simulink model "Tetris"  (R2023a)
settings: Solver=VariableStepAuto  StartTime=0.0  StopTime=inf  RelTol=1e-3  EnableMultiTasking=on
libraries: Miscellaneous x183, Byte_Multiplexers_Lib x77, Tetris_Lib x34, simulink_extras x11, Counters_Lib x7, Arithmetic_Operations_Lib x5, Word_Multiplexers_Lib x5, Decoders_Lib x4, Memory_Blocks_Lib x3, Bit_Multiplexers_Lib x2, dspobslib x1
(part 2 of 3)

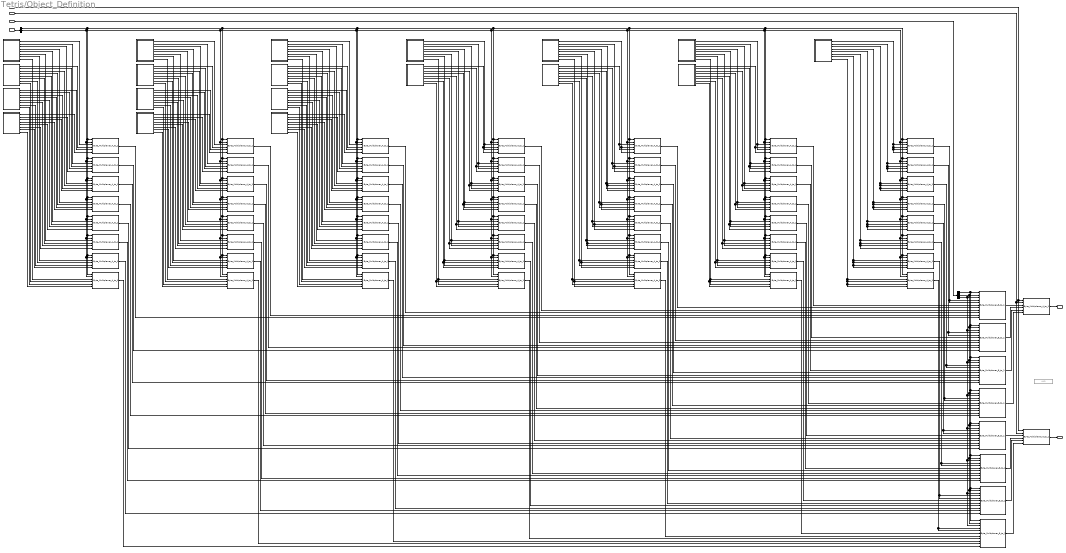
== system Tetris/Object_Definition ==
  Addr_1(1b) : Inport
  Addr_0(1b) : Inport  Port=2
  Shape(1B) : Inport  Port=3
  Angle(1B) : Inport  Port=4
  Bus Selector1 : BusSelector  OutputSignals=signal6,signal7,signal8
  Bus Selector2 : BusSelector  OutputSignals=signal7,signal8
  Byte_Multiplexer_4_to_1(X) : Byte_Multiplexers_Lib/Byte_Multiplexers_Lib/Byte_Multiplexer_4_to_1  SystemSampleTime=-1  VariantActivationTime=update diagram  Latency=0  AutoFrameSizeCalculation=off
  Byte_Multiplexer_4_to_1(Y) : Byte_Multiplexers_Lib/Byte_Multiplexers_Lib/Byte_Multiplexer_4_to_1  SystemSampleTime=-1  VariantActivationTime=update diagram  Latency=0  AutoFrameSizeCalculation=off
  I-shape (0deg) : Subsystem
  I-shape (90deg) : Subsystem
  L1-shape (0deg) : Subsystem
  L1-shape (180deg) : Subsystem
  L1-shape (270deg) : Subsystem
  L1-shape (90deg) : Subsystem
  L2-shape (0deg) : Subsystem
  L2-shape (180deg) : Subsystem
  L2-shape (270deg) : Subsystem
  L2-shape (90deg) : Subsystem
  Logical Operator1 : Logic  Commented=on  Inputs=12  IconShape=distinctive  AllPortsSameDT=off  OutDataTypeStr=boolean
  O-shape : Subsystem
  Select_Angle_I(X0) : Byte_Multiplexers_Lib/Byte_Multiplexers_Lib/Byte_Multiplexer_4_to_1  SystemSampleTime=-1  VariantActivationTime=update diagram  Latency=0  AutoFrameSizeCalculation=off
  Select_Angle_I(X1) : Byte_Multiplexers_Lib/Byte_Multiplexers_Lib/Byte_Multiplexer_4_to_1  SystemSampleTime=-1  VariantActivationTime=update diagram  Latency=0  AutoFrameSizeCalculation=off
  Select_Angle_I(X2) : Byte_Multiplexers_Lib/Byte_Multiplexers_Lib/Byte_Multiplexer_4_to_1  SystemSampleTime=-1  VariantActivationTime=update diagram  Latency=0  AutoFrameSizeCalculation=off
  Select_Angle_I(X3) : Byte_Multiplexers_Lib/Byte_Multiplexers_Lib/Byte_Multiplexer_4_to_1  SystemSampleTime=-1  VariantActivationTime=update diagram  Latency=0  AutoFrameSizeCalculation=off
  Select_Angle_I(Y0) : Byte_Multiplexers_Lib/Byte_Multiplexers_Lib/Byte_Multiplexer_4_to_1  SystemSampleTime=-1  VariantActivationTime=update diagram  Latency=0  AutoFrameSizeCalculation=off
  Select_Angle_I(Y1) : Byte_Multiplexers_Lib/Byte_Multiplexers_Lib/Byte_Multiplexer_4_to_1  SystemSampleTime=-1  VariantActivationTime=update diagram  Latency=0  AutoFrameSizeCalculation=off
  Select_Angle_I(Y2) : Byte_Multiplexers_Lib/Byte_Multiplexers_Lib/Byte_Multiplexer_4_to_1  SystemSampleTime=-1  VariantActivationTime=update diagram  Latency=0  AutoFrameSizeCalculation=off
  Select_Angle_I(Y3) : Byte_Multiplexers_Lib/Byte_Multiplexers_Lib/Byte_Multiplexer_4_to_1  SystemSampleTime=-1  VariantActivationTime=update diagram  Latency=0  AutoFrameSizeCalculation=off
  Select_Angle_L1(X0) : Byte_Multiplexers_Lib/Byte_Multiplexers_Lib/Byte_Multiplexer_4_to_1  SystemSampleTime=-1  VariantActivationTime=update diagram  Latency=0  AutoFrameSizeCalculation=off
  Select_Angle_L1(X1) : Byte_Multiplexers_Lib/Byte_Multiplexers_Lib/Byte_Multiplexer_4_to_1  SystemSampleTime=-1  VariantActivationTime=update diagram  Latency=0  AutoFrameSizeCalculation=off
  Select_Angle_L1(X2) : Byte_Multiplexers_Lib/Byte_Multiplexers_Lib/Byte_Multiplexer_4_to_1  SystemSampleTime=-1  VariantActivationTime=update diagram  Latency=0  AutoFrameSizeCalculation=off
  Select_Angle_L1(X3) : Byte_Multiplexers_Lib/Byte_Multiplexers_Lib/Byte_Multiplexer_4_to_1  SystemSampleTime=-1  VariantActivationTime=update diagram  Latency=0  AutoFrameSizeCalculation=off
  Select_Angle_L1(Y0) : Byte_Multiplexers_Lib/Byte_Multiplexers_Lib/Byte_Multiplexer_4_to_1  SystemSampleTime=-1  VariantActivationTime=update diagram  Latency=0  AutoFrameSizeCalculation=off
  Select_Angle_L1(Y1) : Byte_Multiplexers_Lib/Byte_Multiplexers_Lib/Byte_Multiplexer_4_to_1  SystemSampleTime=-1  VariantActivationTime=update diagram  Latency=0  AutoFrameSizeCalculation=off
  Select_Angle_L1(Y2) : Byte_Multiplexers_Lib/Byte_Multiplexers_Lib/Byte_Multiplexer_4_to_1  SystemSampleTime=-1  VariantActivationTime=update diagram  Latency=0  AutoFrameSizeCalculation=off
  Select_Angle_L1(Y3) : Byte_Multiplexers_Lib/Byte_Multiplexers_Lib/Byte_Multiplexer_4_to_1  SystemSampleTime=-1  VariantActivationTime=update diagram  Latency=0  AutoFrameSizeCalculation=off
  Select_Angle_L2(X0) : Byte_Multiplexers_Lib/Byte_Multiplexers_Lib/Byte_Multiplexer_4_to_1  SystemSampleTime=-1  VariantActivationTime=update diagram  Latency=0  AutoFrameSizeCalculation=off
  Select_Angle_L2(X1) : Byte_Multiplexers_Lib/Byte_Multiplexers_Lib/Byte_Multiplexer_4_to_1  SystemSampleTime=-1  VariantActivationTime=update diagram  Latency=0  AutoFrameSizeCalculation=off
  Select_Angle_L2(X2) : Byte_Multiplexers_Lib/Byte_Multiplexers_Lib/Byte_Multiplexer_4_to_1  SystemSampleTime=-1  VariantActivationTime=update diagram  Latency=0  AutoFrameSizeCalculation=off
  Select_Angle_L2(X3) : Byte_Multiplexers_Lib/Byte_Multiplexers_Lib/Byte_Multiplexer_4_to_1  SystemSampleTime=-1  VariantActivationTime=update diagram  Latency=0  AutoFrameSizeCalculation=off
  Select_Angle_L2(Y0) : Byte_Multiplexers_Lib/Byte_Multiplexers_Lib/Byte_Multiplexer_4_to_1  SystemSampleTime=-1  VariantActivationTime=update diagram  Latency=0  AutoFrameSizeCalculation=off
  Select_Angle_L2(Y1) : Byte_Multiplexers_Lib/Byte_Multiplexers_Lib/Byte_Multiplexer_4_to_1  SystemSampleTime=-1  VariantActivationTime=update diagram  Latency=0  AutoFrameSizeCalculation=off
  Select_Angle_L2(Y2) : Byte_Multiplexers_Lib/Byte_Multiplexers_Lib/Byte_Multiplexer_4_to_1  SystemSampleTime=-1  VariantActivationTime=update diagram  Latency=0  AutoFrameSizeCalculation=off
  Select_Angle_L2(Y3) : Byte_Multiplexers_Lib/Byte_Multiplexers_Lib/Byte_Multiplexer_4_to_1  SystemSampleTime=-1  VariantActivationTime=update diagram  Latency=0  AutoFrameSizeCalculation=off
  Select_Angle_O(X0) : Byte_Multiplexers_Lib/Byte_Multiplexers_Lib/Byte_Multiplexer_4_to_1  SystemSampleTime=-1  VariantActivationTime=update diagram  Latency=0  AutoFrameSizeCalculation=off
  Select_Angle_O(X1) : Byte_Multiplexers_Lib/Byte_Multiplexers_Lib/Byte_Multiplexer_4_to_1  SystemSampleTime=-1  VariantActivationTime=update diagram  Latency=0  AutoFrameSizeCalculation=off
  Select_Angle_O(X2) : Byte_Multiplexers_Lib/Byte_Multiplexers_Lib/Byte_Multiplexer_4_to_1  SystemSampleTime=-1  VariantActivationTime=update diagram  Latency=0  AutoFrameSizeCalculation=off
  Select_Angle_O(X3) : Byte_Multiplexers_Lib/Byte_Multiplexers_Lib/Byte_Multiplexer_4_to_1  SystemSampleTime=-1  VariantActivationTime=update diagram  Latency=0  AutoFrameSizeCalculation=off
  Select_Angle_O(Y0) : Byte_Multiplexers_Lib/Byte_Multiplexers_Lib/Byte_Multiplexer_4_to_1  SystemSampleTime=-1  VariantActivationTime=update diagram  Latency=0  AutoFrameSizeCalculation=off
  Select_Angle_O(Y1) : Byte_Multiplexers_Lib/Byte_Multiplexers_Lib/Byte_Multiplexer_4_to_1  SystemSampleTime=-1  VariantActivationTime=update diagram  Latency=0  AutoFrameSizeCalculation=off
  Select_Angle_O(Y2) : Byte_Multiplexers_Lib/Byte_Multiplexers_Lib/Byte_Multiplexer_4_to_1  SystemSampleTime=-1  VariantActivationTime=update diagram  Latency=0  AutoFrameSizeCalculation=off
  Select_Angle_O(Y3) : Byte_Multiplexers_Lib/Byte_Multiplexers_Lib/Byte_Multiplexer_4_to_1  SystemSampleTime=-1  VariantActivationTime=update diagram  Latency=0  AutoFrameSizeCalculation=off
  Select_Angle_T(X0) : Byte_Multiplexers_Lib/Byte_Multiplexers_Lib/Byte_Multiplexer_4_to_1  SystemSampleTime=-1  VariantActivationTime=update diagram  Latency=0  AutoFrameSizeCalculation=off
  Select_Angle_T(X1) : Byte_Multiplexers_Lib/Byte_Multiplexers_Lib/Byte_Multiplexer_4_to_1  SystemSampleTime=-1  VariantActivationTime=update diagram  Latency=0  AutoFrameSizeCalculation=off
  Select_Angle_T(X2) : Byte_Multiplexers_Lib/Byte_Multiplexers_Lib/Byte_Multiplexer_4_to_1  SystemSampleTime=-1  VariantActivationTime=update diagram  Latency=0  AutoFrameSizeCalculation=off
  Select_Angle_T(X3) : Byte_Multiplexers_Lib/Byte_Multiplexers_Lib/Byte_Multiplexer_4_to_1  SystemSampleTime=-1  VariantActivationTime=update diagram  Latency=0  AutoFrameSizeCalculation=off
  Select_Angle_T(Y0) : Byte_Multiplexers_Lib/Byte_Multiplexers_Lib/Byte_Multiplexer_4_to_1  SystemSampleTime=-1  VariantActivationTime=update diagram  Latency=0  AutoFrameSizeCalculation=off
  Select_Angle_T(Y1) : Byte_Multiplexers_Lib/Byte_Multiplexers_Lib/Byte_Multiplexer_4_to_1  SystemSampleTime=-1  VariantActivationTime=update diagram  Latency=0  AutoFrameSizeCalculation=off
  Select_Angle_T(Y2) : Byte_Multiplexers_Lib/Byte_Multiplexers_Lib/Byte_Multiplexer_4_to_1  SystemSampleTime=-1  VariantActivationTime=update diagram  Latency=0  AutoFrameSizeCalculation=off
  Select_Angle_T(Y3) : Byte_Multiplexers_Lib/Byte_Multiplexers_Lib/Byte_Multiplexer_4_to_1  SystemSampleTime=-1  VariantActivationTime=update diagram  Latency=0  AutoFrameSizeCalculation=off
  Select_Angle_Z1(X0) : Byte_Multiplexers_Lib/Byte_Multiplexers_Lib/Byte_Multiplexer_4_to_1  SystemSampleTime=-1  VariantActivationTime=update diagram  Latency=0  AutoFrameSizeCalculation=off
  Select_Angle_Z1(X1) : Byte_Multiplexers_Lib/Byte_Multiplexers_Lib/Byte_Multiplexer_4_to_1  SystemSampleTime=-1  VariantActivationTime=update diagram  Latency=0  AutoFrameSizeCalculation=off
  Select_Angle_Z1(X2) : Byte_Multiplexers_Lib/Byte_Multiplexers_Lib/Byte_Multiplexer_4_to_1  SystemSampleTime=-1  VariantActivationTime=update diagram  Latency=0  AutoFrameSizeCalculation=off
  Select_Angle_Z1(X3) : Byte_Multiplexers_Lib/Byte_Multiplexers_Lib/Byte_Multiplexer_4_to_1  SystemSampleTime=-1  VariantActivationTime=update diagram  Latency=0  AutoFrameSizeCalculation=off
  Select_Angle_Z1(Y0) : Byte_Multiplexers_Lib/Byte_Multiplexers_Lib/Byte_Multiplexer_4_to_1  SystemSampleTime=-1  VariantActivationTime=update diagram  Latency=0  AutoFrameSizeCalculation=off
  Select_Angle_Z1(Y1) : Byte_Multiplexers_Lib/Byte_Multiplexers_Lib/Byte_Multiplexer_4_to_1  SystemSampleTime=-1  VariantActivationTime=update diagram  Latency=0  AutoFrameSizeCalculation=off
  Select_Angle_Z1(Y2) : Byte_Multiplexers_Lib/Byte_Multiplexers_Lib/Byte_Multiplexer_4_to_1  SystemSampleTime=-1  VariantActivationTime=update diagram  Latency=0  AutoFrameSizeCalculation=off
  Select_Angle_Z1(Y3) : Byte_Multiplexers_Lib/Byte_Multiplexers_Lib/Byte_Multiplexer_4_to_1  SystemSampleTime=-1  VariantActivationTime=update diagram  Latency=0  AutoFrameSizeCalculation=off
  Select_Angle_Z2(X0) : Byte_Multiplexers_Lib/Byte_Multiplexers_Lib/Byte_Multiplexer_4_to_1  SystemSampleTime=-1  VariantActivationTime=update diagram  Latency=0  AutoFrameSizeCalculation=off
  Select_Angle_Z2(X1) : Byte_Multiplexers_Lib/Byte_Multiplexers_Lib/Byte_Multiplexer_4_to_1  SystemSampleTime=-1  VariantActivationTime=update diagram  Latency=0  AutoFrameSizeCalculation=off
  Select_Angle_Z2(X2) : Byte_Multiplexers_Lib/Byte_Multiplexers_Lib/Byte_Multiplexer_4_to_1  SystemSampleTime=-1  VariantActivationTime=update diagram  Latency=0  AutoFrameSizeCalculation=off
  Select_Angle_Z2(X3) : Byte_Multiplexers_Lib/Byte_Multiplexers_Lib/Byte_Multiplexer_4_to_1  SystemSampleTime=-1  VariantActivationTime=update diagram  Latency=0  AutoFrameSizeCalculation=off
  Select_Angle_Z2(Y0) : Byte_Multiplexers_Lib/Byte_Multiplexers_Lib/Byte_Multiplexer_4_to_1  SystemSampleTime=-1  VariantActivationTime=update diagram  Latency=0  AutoFrameSizeCalculation=off
  Select_Angle_Z2(Y1) : Byte_Multiplexers_Lib/Byte_Multiplexers_Lib/Byte_Multiplexer_4_to_1  SystemSampleTime=-1  VariantActivationTime=update diagram  Latency=0  AutoFrameSizeCalculation=off
  Select_Angle_Z2(Y2) : Byte_Multiplexers_Lib/Byte_Multiplexers_Lib/Byte_Multiplexer_4_to_1  SystemSampleTime=-1  VariantActivationTime=update diagram  Latency=0  AutoFrameSizeCalculation=off
  Select_Angle_Z2(Y3) : Byte_Multiplexers_Lib/Byte_Multiplexers_Lib/Byte_Multiplexer_4_to_1  SystemSampleTime=-1  VariantActivationTime=update diagram  Latency=0  AutoFrameSizeCalculation=off
  Select_Shape(X0) : Byte_Multiplexers_Lib/Byte_Multiplexers_Lib/Byte_Multiplexer_8_to_1  SystemSampleTime=-1  VariantActivationTime=update diagram  Latency=0  AutoFrameSizeCalculation=off
  Select_Shape(X1) : Byte_Multiplexers_Lib/Byte_Multiplexers_Lib/Byte_Multiplexer_8_to_1  SystemSampleTime=-1  VariantActivationTime=update diagram  Latency=0  AutoFrameSizeCalculation=off
  Select_Shape(X2) : Byte_Multiplexers_Lib/Byte_Multiplexers_Lib/Byte_Multiplexer_8_to_1  SystemSampleTime=-1  VariantActivationTime=update diagram  Latency=0  AutoFrameSizeCalculation=off
  Select_Shape(X3) : Byte_Multiplexers_Lib/Byte_Multiplexers_Lib/Byte_Multiplexer_8_to_1  SystemSampleTime=-1  VariantActivationTime=update diagram  Latency=0  AutoFrameSizeCalculation=off
  Select_Shape(Y0) : Byte_Multiplexers_Lib/Byte_Multiplexers_Lib/Byte_Multiplexer_8_to_1  SystemSampleTime=-1  VariantActivationTime=update diagram  Latency=0  AutoFrameSizeCalculation=off
  Select_Shape(Y1) : Byte_Multiplexers_Lib/Byte_Multiplexers_Lib/Byte_Multiplexer_8_to_1  SystemSampleTime=-1  VariantActivationTime=update diagram  Latency=0  AutoFrameSizeCalculation=off
  Select_Shape(Y2) : Byte_Multiplexers_Lib/Byte_Multiplexers_Lib/Byte_Multiplexer_8_to_1  SystemSampleTime=-1  VariantActivationTime=update diagram  Latency=0  AutoFrameSizeCalculation=off
  Select_Shape(Y3) : Byte_Multiplexers_Lib/Byte_Multiplexers_Lib/Byte_Multiplexer_8_to_1  SystemSampleTime=-1  VariantActivationTime=update diagram  Latency=0  AutoFrameSizeCalculation=off
  T-shape (0deg) : Subsystem
  T-shape (180deg) : Subsystem
  T-shape (270deg) : Subsystem
  T-shape (90deg) : Subsystem
  Z1-shape (0deg) : Subsystem
  Z1-shape (90deg) : Subsystem
  Z2-shape (0deg) : Subsystem
  Z2-shape (90deg) : Subsystem
  X(1B) : Outport
  Y(1B) : Outport  Port=2
  wires:
  L2-shape (0deg)/1(X0(1B)) -> Select_Angle_L2(X3)/3
  L2-shape (90deg)/1(X0(1B)) -> Select_Angle_L2(X3)/4
  L2-shape (180deg)/1(X0(1B)) -> Select_Angle_L2(X3)/5
  L2-shape (270deg)/1(X0(1B)) -> Select_Angle_L2(X3)/6
  L2-shape (0deg)/2(X1(1B)) -> Select_Angle_L2(X2)/3
  L2-shape (90deg)/2(X1(1B)) -> Select_Angle_L2(X2)/4
  L2-shape (180deg)/2(X1(1B)) -> Select_Angle_L2(X2)/5
  L2-shape (270deg)/2(X1(1B)) -> Select_Angle_L2(X2)/6
  L2-shape (0deg)/3(X2(1B)) -> Select_Angle_L2(X1)/3
  L2-shape (90deg)/3(X2(1B)) -> Select_Angle_L2(X1)/4
  L2-shape (180deg)/3(X2(1B)) -> Select_Angle_L2(X1)/5
  L2-shape (270deg)/3(X2(1B)) -> Select_Angle_L2(X1)/6
  L2-shape (0deg)/4(X3(1B)) -> Select_Angle_L2(X0)/3
  L2-shape (90deg)/4(X3(1B)) -> Select_Angle_L2(X0)/4
  L2-shape (180deg)/4(X3(1B)) -> Select_Angle_L2(X0)/5
  L2-shape (270deg)/4(X3(1B)) -> Select_Angle_L2(X0)/6
  L2-shape (0deg)/5(Y0(1B)) -> Select_Angle_L2(Y3)/3
  L2-shape (90deg)/5(Y0(1B)) -> Select_Angle_L2(Y3)/4
  L2-shape (180deg)/5(Y0(1B)) -> Select_Angle_L2(Y3)/5
  L2-shape (270deg)/5(Y0(1B)) -> Select_Angle_L2(Y3)/6
  L2-shape (0deg)/6(Y1(1B)) -> Select_Angle_L2(Y2)/3
  L2-shape (90deg)/6(Y1(1B)) -> Select_Angle_L2(Y2)/4
  L2-shape (180deg)/6(Y1(1B)) -> Select_Angle_L2(Y2)/5
  L2-shape (270deg)/6(Y1(1B)) -> Select_Angle_L2(Y2)/6
  L2-shape (0deg)/7(Y2(1B)) -> Select_Angle_L2(Y1)/3
  L2-shape (90deg)/7(Y2(1B)) -> Select_Angle_L2(Y1)/4
  L2-shape (180deg)/7(Y2(1B)) -> Select_Angle_L2(Y1)/5
  L2-shape (270deg)/7(Y2(1B)) -> Select_Angle_L2(Y1)/6
  L2-shape (0deg)/8(Y3(1B)) -> Select_Angle_L2(Y0)/3
  L2-shape (90deg)/8(Y3(1B)) -> Select_Angle_L2(Y0)/4
  L2-shape (180deg)/8(Y3(1B)) -> Select_Angle_L2(Y0)/5
  L2-shape (270deg)/8(Y3(1B)) -> Select_Angle_L2(Y0)/6
  Angle(1B)/1 -> Bus Selector2/1
  L1-shape (270deg)/4(X3(1B)) -> Select_Angle_L1(X0)/6
  L1-shape (180deg)/4(X3(1B)) -> Select_Angle_L1(X0)/5
  L1-shape (270deg)/6(Y1(1B)) -> Select_Angle_L1(Y2)/6
  L1-shape (180deg)/5(Y0(1B)) -> Select_Angle_L1(Y3)/5
  L1-shape (90deg)/8(Y3(1B)) -> Select_Angle_L1(Y0)/4
  L1-shape (180deg)/1(X0(1B)) -> Select_Angle_L1(X3)/5
  L1-shape (270deg)/5(Y0(1B)) -> Select_Angle_L1(Y3)/6
  L1-shape (90deg)/6(Y1(1B)) -> Select_Angle_L1(Y2)/4
  L1-shape (0deg)/2(X1(1B)) -> Select_Angle_L1(X2)/3
  L1-shape (90deg)/2(X1(1B)) -> Select_Angle_L1(X2)/4
  L1-shape (270deg)/8(Y3(1B)) -> Select_Angle_L1(Y0)/6
  L1-shape (180deg)/6(Y1(1B)) -> Select_Angle_L1(Y2)/5
  L1-shape (0deg)/6(Y1(1B)) -> Select_Angle_L1(Y2)/3
  L1-shape (90deg)/7(Y2(1B)) -> Select_Angle_L1(Y1)/4
  L1-shape (90deg)/3(X2(1B)) -> Select_Angle_L1(X1)/4
  L1-shape (180deg)/3(X2(1B)) -> Select_Angle_L1(X1)/5
  L1-shape (0deg)/1(X0(1B)) -> Select_Angle_L1(X3)/3
  L1-shape (0deg)/7(Y2(1B)) -> Select_Angle_L1(Y1)/3
  L1-shape (0deg)/3(X2(1B)) -> Select_Angle_L1(X1)/3
  L1-shape (0deg)/4(X3(1B)) -> Select_Angle_L1(X0)/3
  L1-shape (270deg)/2(X1(1B)) -> Select_Angle_L1(X2)/6
  L1-shape (90deg)/5(Y0(1B)) -> Select_Angle_L1(Y3)/4
  L1-shape (180deg)/7(Y2(1B)) -> Select_Angle_L1(Y1)/5
  L1-shape (90deg)/1(X0(1B)) -> Select_Angle_L1(X3)/4
  L1-shape (180deg)/8(Y3(1B)) -> Select_Angle_L1(Y0)/5
  L1-shape (270deg)/7(Y2(1B)) -> Select_Angle_L1(Y1)/6
  L1-shape (270deg)/1(X0(1B)) -> Select_Angle_L1(X3)/6
  L1-shape (0deg)/5(Y0(1B)) -> Select_Angle_L1(Y3)/3
  L1-shape (270deg)/3(X2(1B)) -> Select_Angle_L1(X1)/6
  L1-shape (180deg)/2(X1(1B)) -> Select_Angle_L1(X2)/5
  L1-shape (0deg)/8(Y3(1B)) -> Select_Angle_L1(Y0)/3
  L1-shape (90deg)/4(X3(1B)) -> Select_Angle_L1(X0)/4
  T-shape (90deg)/1(X0(1B)) -> Select_Angle_T(X3)/4
  T-shape (90deg)/5(Y0(1B)) -> Select_Angle_T(Y3)/4
  T-shape (90deg)/7(Y2(1B)) -> Select_Angle_T(Y1)/4
  T-shape (90deg)/6(Y1(1B)) -> Select_Angle_T(Y2)/4
  T-shape (180deg)/8(Y3(1B)) -> Select_Angle_T(Y0)/5
  T-shape (180deg)/6(Y1(1B)) -> Select_Angle_T(Y2)/5
  T-shape (90deg)/4(X3(1B)) -> Select_Angle_T(X0)/4
  T-shape (180deg)/7(Y2(1B)) -> Select_Angle_T(Y1)/5
  T-shape (180deg)/4(X3(1B)) -> Select_Angle_T(X0)/5
  T-shape (180deg)/1(X0(1B)) -> Select_Angle_T(X3)/5
  T-shape (180deg)/3(X2(1B)) -> Select_Angle_T(X1)/5
  T-shape (90deg)/2(X1(1B)) -> Select_Angle_T(X2)/4
  T-shape (180deg)/5(Y0(1B)) -> Select_Angle_T(Y3)/5
  T-shape (270deg)/1(X0(1B)) -> Select_Angle_T(X3)/6
  T-shape (270deg)/5(Y0(1B)) -> Select_Angle_T(Y3)/6
  T-shape (270deg)/7(Y2(1B)) -> Select_Angle_T(Y1)/6
  T-shape (270deg)/4(X3(1B)) -> Select_Angle_T(X0)/6
  T-shape (270deg)/3(X2(1B)) -> Select_Angle_T(X1)/6
  T-shape (270deg)/2(X1(1B)) -> Select_Angle_T(X2)/6
  T-shape (270deg)/8(Y3(1B)) -> Select_Angle_T(Y0)/6
  T-shape (270deg)/6(Y1(1B)) -> Select_Angle_T(Y2)/6
  T-shape (0deg)/1(X0(1B)) -> Select_Angle_T(X3)/3
  T-shape (180deg)/2(X1(1B)) -> Select_Angle_T(X2)/5
  T-shape (0deg)/8(Y3(1B)) -> Select_Angle_T(Y0)/3
  T-shape (90deg)/8(Y3(1B)) -> Select_Angle_T(Y0)/4
  T-shape (0deg)/6(Y1(1B)) -> Select_Angle_T(Y2)/3
  T-shape (0deg)/3(X2(1B)) -> Select_Angle_T(X1)/3
  T-shape (0deg)/4(X3(1B)) -> Select_Angle_T(X0)/3
  T-shape (90deg)/3(X2(1B)) -> Select_Angle_T(X1)/4
  T-shape (0deg)/2(X1(1B)) -> Select_Angle_T(X2)/3
  T-shape (0deg)/5(Y0(1B)) -> Select_Angle_T(Y3)/3
  T-shape (0deg)/7(Y2(1B)) -> Select_Angle_T(Y1)/3
  Z2-shape (0deg)/8(Y3(1B)) -> Select_Angle_Z2(Y0)/5, Select_Angle_Z2(Y0)/3
  Z2-shape (0deg)/6(Y1(1B)) -> Select_Angle_Z2(Y2)/5, Select_Angle_Z2(Y2)/3
  Z2-shape (0deg)/7(Y2(1B)) -> Select_Angle_Z2(Y1)/5, Select_Angle_Z2(Y1)/3
  Z2-shape (0deg)/4(X3(1B)) -> Select_Angle_Z2(X0)/5, Select_Angle_Z2(X0)/3
  Z2-shape (0deg)/1(X0(1B)) -> Select_Angle_Z2(X3)/5, Select_Angle_Z2(X3)/3
  Z2-shape (0deg)/3(X2(1B)) -> Select_Angle_Z2(X1)/5, Select_Angle_Z2(X1)/3
  Z2-shape (0deg)/5(Y0(1B)) -> Select_Angle_Z2(Y3)/5, Select_Angle_Z2(Y3)/3
  Z2-shape (90deg)/1(X0(1B)) -> Select_Angle_Z2(X3)/6, Select_Angle_Z2(X3)/4
  Z2-shape (90deg)/5(Y0(1B)) -> Select_Angle_Z2(Y3)/6, Select_Angle_Z2(Y3)/4
  Z2-shape (90deg)/7(Y2(1B)) -> Select_Angle_Z2(Y1)/6, Select_Angle_Z2(Y1)/4
  Z2-shape (90deg)/4(X3(1B)) -> Select_Angle_Z2(X0)/6, Select_Angle_Z2(X0)/4
  Z2-shape (90deg)/3(X2(1B)) -> Select_Angle_Z2(X1)/6, Select_Angle_Z2(X1)/4
  Z2-shape (90deg)/2(X1(1B)) -> Select_Angle_Z2(X2)/6, Select_Angle_Z2(X2)/4
  Z2-shape (90deg)/8(Y3(1B)) -> Select_Angle_Z2(Y0)/6, Select_Angle_Z2(Y0)/4
  Z2-shape (90deg)/6(Y1(1B)) -> Select_Angle_Z2(Y2)/6, Select_Angle_Z2(Y2)/4
  Z2-shape (0deg)/2(X1(1B)) -> Select_Angle_Z2(X2)/5, Select_Angle_Z2(X2)/3
  Z1-shape (90deg)/7(Y1(1B)) -> Select_Angle_Z1(Y1)/5, Select_Angle_Z1(Y1)/3
  Z1-shape (90deg)/2(X2(1B)) -> Select_Angle_Z1(X2)/5, Select_Angle_Z1(X2)/3
  Z1-shape (90deg)/4(X0(1B)) -> Select_Angle_Z1(X0)/5, Select_Angle_Z1(X0)/3
  Z1-shape (90deg)/3(X1(1B)) -> Select_Angle_Z1(X1)/5, Select_Angle_Z1(X1)/3
  Z1-shape (90deg)/6(Y2(1B)) -> Select_Angle_Z1(Y2)/5, Select_Angle_Z1(Y2)/3
  Z1-shape (90deg)/5(Y3(1B)) -> Select_Angle_Z1(Y3)/5, Select_Angle_Z1(Y3)/3
  Z1-shape (90deg)/1(X3(1B)) -> Select_Angle_Z1(X3)/5, Select_Angle_Z1(X3)/3
  Z1-shape (0deg)/6(Y2(1B)) -> Select_Angle_Z1(Y2)/6, Select_Angle_Z1(Y2)/4
  Z1-shape (0deg)/4(X0(1B)) -> Select_Angle_Z1(X0)/6, Select_Angle_Z1(X0)/4
  Z1-shape (0deg)/1(X3(1B)) -> Select_Angle_Z1(X3)/6, Select_Angle_Z1(X3)/4
  Z1-shape (0deg)/5(Y3(1B)) -> Select_Angle_Z1(Y3)/6, Select_Angle_Z1(Y3)/4
  Z1-shape (90deg)/8(Y0(1B)) -> Select_Angle_Z1(Y0)/5, Select_Angle_Z1(Y0)/3
  Z1-shape (0deg)/2(X2(1B)) -> Select_Angle_Z1(X2)/4, Select_Angle_Z1(X2)/6
  Z1-shape (0deg)/3(X1(1B)) -> Select_Angle_Z1(X1)/6, Select_Angle_Z1(X1)/4
  Z1-shape (0deg)/8(Y0(1B)) -> Select_Angle_Z1(Y0)/6, Select_Angle_Z1(Y0)/4
  Z1-shape (0deg)/7(Y1(1B)) -> Select_Angle_Z1(Y1)/6, Select_Angle_Z1(Y1)/4
  I-shape (90deg)/7(Y2(1B)) -> Select_Angle_I(Y1)/6, Select_Angle_I(Y1)/4
  I-shape (90deg)/2(X1(1B)) -> Select_Angle_I(X2)/6, Select_Angle_I(X2)/4
  I-shape (90deg)/4(X3(1B)) -> Select_Angle_I(X0)/6, Select_Angle_I(X0)/4
  I-shape (90deg)/3(X2(1B)) -> Select_Angle_I(X1)/6, Select_Angle_I(X1)/4
  I-shape (90deg)/6(Y1(1B)) -> Select_Angle_I(Y2)/6, Select_Angle_I(Y2)/4
  I-shape (90deg)/5(Y0(1B)) -> Select_Angle_I(Y3)/6, Select_Angle_I(Y3)/4
  I-shape (90deg)/1(X0(1B)) -> Select_Angle_I(X3)/6, Select_Angle_I(X3)/4
  I-shape (0deg)/6(Y1(1B)) -> Select_Angle_I(Y2)/5, Select_Angle_I(Y2)/3
  I-shape (0deg)/4(X3(1B)) -> Select_Angle_I(X0)/5, Select_Angle_I(X0)/3
  I-shape (0deg)/1(X0(1B)) -> Select_Angle_I(X3)/5, Select_Angle_I(X3)/3
  I-shape (0deg)/5(Y0(1B)) -> Select_Angle_I(Y3)/5, Select_Angle_I(Y3)/3
  I-shape (90deg)/8(Y3(1B)) -> Select_Angle_I(Y0)/6, Select_Angle_I(Y0)/4
  I-shape (0deg)/2(X1(1B)) -> Select_Angle_I(X2)/5, Select_Angle_I(X2)/3
  I-shape (0deg)/3(X2(1B)) -> Select_Angle_I(X1)/5, Select_Angle_I(X1)/3
  I-shape (0deg)/8(Y3(1B)) -> Select_Angle_I(Y0)/5, Select_Angle_I(Y0)/3
  I-shape (0deg)/7(Y2(1B)) -> Select_Angle_I(Y1)/5, Select_Angle_I(Y1)/3
  O-shape/7(Y2(1B)) -> Select_Angle_O(Y1)/5, Select_Angle_O(Y1)/6, Select_Angle_O(Y1)/4, Select_Angle_O(Y1)/3
  O-shape/2(X1(1B)) -> Select_Angle_O(X2)/5, Select_Angle_O(X2)/6, Select_Angle_O(X2)/4, Select_Angle_O(X2)/3
  O-shape/4(X3(1B)) -> Select_Angle_O(X0)/5, Select_Angle_O(X0)/6, Select_Angle_O(X0)/4, Select_Angle_O(X0)/3
  O-shape/3(X2(1B)) -> Select_Angle_O(X1)/5, Select_Angle_O(X1)/6, Select_Angle_O(X1)/4, Select_Angle_O(X1)/3
  O-shape/6(Y1(1B)) -> Select_Angle_O(Y2)/6, Select_Angle_O(Y2)/5, Select_Angle_O(Y2)/4, Select_Angle_O(Y2)/3
  O-shape/5(Y0(1B)) -> Select_Angle_O(Y3)/5, Select_Angle_O(Y3)/6, Select_Angle_O(Y3)/4, Select_Angle_O(Y3)/3
  O-shape/1(X0(1B)) -> Select_Angle_O(X3)/5, Select_Angle_O(X3)/6, Select_Angle_O(X3)/4, Select_Angle_O(X3)/3
  Bus Selector2/1 -> Select_Angle_L2(Y0)/1, Select_Angle_L2(Y1)/1, Select_Angle_L2(Y2)/1, Select_Angle_L2(Y3)/1, Select_Angle_L2(X0)/1, Select_Angle_L2(X1)/1, Select_Angle_L2(X2)/1, Select_Angle_L2(X3)/1, Select_Angle_Z1(Y0)/1, Select_Angle_Z1(Y1)/1, Select_Angle_Z1(Y2)/1, Select_Angle_Z1(Y3)/1, Select_Angle_Z1(X0)/1, Select_Angle_Z1(X1)/1, Select_Angle_Z1(X2)/1, Select_Angle_Z1(X3)/1, Select_Angle_O(Y0)/1, Select_Angle_O(Y1)/1, Select_Angle_O(Y2)/1, Select_Angle_O(Y3)/1, Select_Angle_O(X0)/1, Select_Angle_O(X1)/1, Select_Angle_O(X2)/1, Select_Angle_O(X3)/1, Select_Angle_I(Y0)/1, Select_Angle_I(Y1)/1, Select_Angle_I(Y2)/1, Select_Angle_I(Y3)/1, Select_Angle_I(X0)/1, Select_Angle_I(X1)/1, Select_Angle_I(X2)/1, Select_Angle_I(X3)/1, Select_Angle_Z2(Y0)/1, Select_Angle_Z2(Y1)/1, Select_Angle_Z2(Y2)/1, Select_Angle_Z2(Y3)/1, Select_Angle_Z2(X0)/1, Select_Angle_Z2(X1)/1, Select_Angle_Z2(X2)/1, Select_Angle_Z2(X3)/1, Select_Angle_T(Y0)/1, Select_Angle_T(Y1)/1, Select_Angle_T(Y2)/1, Select_Angle_T(Y3)/1, Select_Angle_T(X0)/1, Select_Angle_T(X1)/1, Select_Angle_T(X2)/1, Select_Angle_T(X3)/1, Select_Angle_L1(Y0)/1, Select_Angle_L1(Y1)/1, Select_Angle_L1(Y2)/1, Select_Angle_L1(Y3)/1, Select_Angle_L1(X0)/1, Select_Angle_L1(X1)/1, Select_Angle_L1(X2)/1, Select_Angle_L1(X3)/1  "<signal7>"
  Bus Selector2/2 -> Select_Angle_L2(Y0)/2, Select_Angle_L2(Y1)/2, Select_Angle_L2(Y2)/2, Select_Angle_L2(Y3)/2, Select_Angle_L2(X0)/2, Select_Angle_L2(X1)/2, Select_Angle_L2(X2)/2, Select_Angle_L2(X3)/2, Select_Angle_Z1(Y0)/2, Select_Angle_Z1(Y1)/2, Select_Angle_Z1(Y2)/2, Select_Angle_Z1(Y3)/2, Select_Angle_Z1(X0)/2, Select_Angle_Z1(X1)/2, Select_Angle_Z1(X2)/2, Select_Angle_Z1(X3)/2, Select_Angle_O(Y0)/2, Select_Angle_O(Y1)/2, Select_Angle_O(Y2)/2, Select_Angle_O(Y3)/2, Select_Angle_O(X0)/2, Select_Angle_O(X1)/2, Select_Angle_O(X2)/2, Select_Angle_O(X3)/2, Select_Angle_I(Y0)/2, Select_Angle_I(Y1)/2, Select_Angle_I(Y2)/2, Select_Angle_I(Y3)/2, Select_Angle_I(X0)/2, Select_Angle_I(X1)/2, Select_Angle_I(X2)/2, Select_Angle_I(X3)/2, Select_Angle_Z2(Y0)/2, Select_Angle_Z2(Y1)/2, Select_Angle_Z2(Y2)/2, Select_Angle_Z2(Y3)/2, Select_Angle_Z2(X0)/2, Select_Angle_Z2(X1)/2, Select_Angle_Z2(X2)/2, Select_Angle_Z2(X3)/2, Select_Angle_T(Y0)/2, Select_Angle_T(Y1)/2, Select_Angle_T(Y2)/2, Select_Angle_T(Y3)/2, Select_Angle_T(X0)/2, Select_Angle_T(X1)/2, Select_Angle_T(X2)/2, Select_Angle_T(X3)/2, Select_Angle_L1(Y0)/2, Select_Angle_L1(Y1)/2, Select_Angle_L1(Y2)/2, Select_Angle_L1(Y3)/2, Select_Angle_L1(X0)/2, Select_Angle_L1(X1)/2, Select_Angle_L1(X2)/2, Select_Angle_L1(X3)/2  "<signal8>"
  O-shape/8(Y3(1B)) -> Select_Angle_O(Y0)/5, Select_Angle_O(Y0)/6, Select_Angle_O(Y0)/4, Select_Angle_O(Y0)/3
  Select_Angle_O(X3)/1 -> Select_Shape(X3)/4, Select_Shape(X3)/5
  Select_Angle_I(X3)/1 -> Select_Shape(X3)/6
  Select_Angle_Z1(X3)/1 -> Select_Shape(X3)/7
  Select_Angle_Z2(X3)/1 -> Select_Shape(X3)/8
  Select_Angle_T(X3)/1 -> Select_Shape(X3)/9
  Select_Angle_L1(X3)/1 -> Select_Shape(X3)/10
  Select_Angle_L2(X3)/1 -> Select_Shape(X3)/11
  Select_Angle_L2(X2)/1 -> Select_Shape(X2)/11
  Select_Angle_L2(X1)/1 -> Select_Shape(X1)/11
  Select_Angle_L2(X0)/1 -> Select_Shape(X0)/11
  Select_Angle_L2(Y3)/1 -> Select_Shape(Y3)/11
  Select_Angle_L2(Y2)/1 -> Select_Shape(Y2)/11
  Select_Angle_L2(Y1)/1 -> Select_Shape(Y1)/11
  Select_Angle_L2(Y0)/1 -> Select_Shape(Y0)/11
  Select_Angle_L1(X2)/1 -> Select_Shape(X2)/10
  Select_Angle_L1(X1)/1 -> Select_Shape(X1)/10
  Select_Angle_L1(X0)/1 -> Select_Shape(X0)/10
  Select_Angle_L1(Y3)/1 -> Select_Shape(Y3)/10
  Select_Angle_L1(Y2)/1 -> Select_Shape(Y2)/10
  Select_Angle_L1(Y1)/1 -> Select_Shape(Y1)/10
  Select_Angle_L1(Y0)/1 -> Select_Shape(Y0)/10
  Select_Angle_T(X2)/1 -> Select_Shape(X2)/9
  Select_Angle_T(X1)/1 -> Select_Shape(X1)/9
  Select_Angle_T(X0)/1 -> Select_Shape(X0)/9
  Select_Angle_T(Y3)/1 -> Select_Shape(Y3)/9
  Select_Angle_T(Y2)/1 -> Select_Shape(Y2)/9
  Select_Angle_T(Y1)/1 -> Select_Shape(Y1)/9
  Select_Angle_T(Y0)/1 -> Select_Shape(Y0)/9
  Select_Angle_Z2(X2)/1 -> Select_Shape(X2)/8
  Select_Angle_Z2(X1)/1 -> Select_Shape(X1)/8
  Select_Angle_Z2(X0)/1 -> Select_Shape(X0)/8
  Select_Angle_Z2(Y3)/1 -> Select_Shape(Y3)/8
  Select_Angle_Z2(Y2)/1 -> Select_Shape(Y2)/8
  Select_Angle_Z2(Y1)/1 -> Select_Shape(Y1)/8
  Select_Angle_Z2(Y0)/1 -> Select_Shape(Y0)/8
  Select_Angle_Z1(X2)/1 -> Select_Shape(X2)/7
  Select_Angle_Z1(X1)/1 -> Select_Shape(X1)/7
  Select_Angle_Z1(X0)/1 -> Select_Shape(X0)/7
  Select_Angle_Z1(Y3)/1 -> Select_Shape(Y3)/7
  Select_Angle_Z1(Y2)/1 -> Select_Shape(Y2)/7
  Select_Angle_Z1(Y1)/1 -> Select_Shape(Y1)/7
  Select_Angle_Z1(Y0)/1 -> Select_Shape(Y0)/7
  Select_Angle_I(X2)/1 -> Select_Shape(X2)/6
  Select_Angle_I(X1)/1 -> Select_Shape(X1)/6
  Select_Angle_I(X0)/1 -> Select_Shape(X0)/6
  Select_Angle_I(Y3)/1 -> Select_Shape(Y3)/6
  Select_Angle_I(Y2)/1 -> Select_Shape(Y2)/6
  Select_Angle_I(Y1)/1 -> Select_Shape(Y1)/6
  Select_Angle_I(Y0)/1 -> Select_Shape(Y0)/6
  Select_Angle_O(X2)/1 -> Select_Shape(X2)/4, Select_Shape(X2)/5
  Select_Angle_O(X1)/1 -> Select_Shape(X1)/4, Select_Shape(X1)/5
  Select_Angle_O(X0)/1 -> Select_Shape(X0)/4, Select_Shape(X0)/5
  Select_Angle_O(Y3)/1 -> Select_Shape(Y3)/4, Select_Shape(Y3)/5
  Select_Angle_O(Y2)/1 -> Select_Shape(Y2)/4, Select_Shape(Y2)/5
  Select_Angle_O(Y1)/1 -> Select_Shape(Y1)/4, Select_Shape(Y1)/5
  Select_Angle_O(Y0)/1 -> Select_Shape(Y0)/4, Select_Shape(Y0)/5
  Shape(1B)/1 -> Bus Selector1/1
  Bus Selector1/1 -> Select_Shape(X3)/1, Select_Shape(X2)/1, Select_Shape(X1)/1, Select_Shape(X0)/1, Select_Shape(Y3)/1, Select_Shape(Y2)/1, Select_Shape(Y1)/1, Select_Shape(Y0)/1  "<signal6>"
  Bus Selector1/2 -> Select_Shape(X3)/2, Select_Shape(X2)/2, Select_Shape(X1)/2, Select_Shape(X0)/2, Select_Shape(Y3)/2, Select_Shape(Y2)/2, Select_Shape(Y1)/2, Select_Shape(Y0)/2  "<signal7>"
  Bus Selector1/3 -> Select_Shape(X3)/3, Select_Shape(X2)/3, Select_Shape(X1)/3, Select_Shape(Y3)/3, Select_Shape(Y2)/3, Select_Shape(Y1)/3, Select_Shape(Y0)/3, Select_Shape(X0)/3  "<signal8>"
  Select_Shape(X3)/1 -> Byte_Multiplexer_4_to_1(X)/3
  Select_Shape(X2)/1 -> Byte_Multiplexer_4_to_1(X)/4
  Select_Shape(X1)/1 -> Byte_Multiplexer_4_to_1(X)/5
  Select_Shape(X0)/1 -> Byte_Multiplexer_4_to_1(X)/6
  Select_Shape(Y3)/1 -> Byte_Multiplexer_4_to_1(Y)/3
  Select_Shape(Y2)/1 -> Byte_Multiplexer_4_to_1(Y)/4
  Select_Shape(Y1)/1 -> Byte_Multiplexer_4_to_1(Y)/5
  Select_Shape(Y0)/1 -> Byte_Multiplexer_4_to_1(Y)/6
  Addr_1(1b)/1 -> Byte_Multiplexer_4_to_1(Y)/1, Byte_Multiplexer_4_to_1(X)/1
  Addr_0(1b)/1 -> Byte_Multiplexer_4_to_1(Y)/2, Byte_Multiplexer_4_to_1(X)/2
  Byte_Multiplexer_4_to_1(X)/1 -> X(1B)/1
  Byte_Multiplexer_4_to_1(Y)/1 -> Y(1B)/1
